simulink model "Lab1"  (Simulink 8.8)
settings: Solver=FixedStepAuto  StartTime=0.0  StopTime=10  FixedStep=0.001  MaxStep=10^-3  RelTol=1e-3  EnableMultiTasking=on
settings Model: Creator=student  LastModifiedBy=Admin
settings OptimizationCC: ExpressionDepthLimit=2147483647  InitFltsAndDblsToZero=on
settings DebuggingCC: SaveWithParameterizedLinksMsg=none  SolverPrmCheckMsg=warning
settings GRTTargetCC: TargetFcnLib=ansi_tfl_tmw.mat  GeneratePreprocessorConditionals=Use local settings

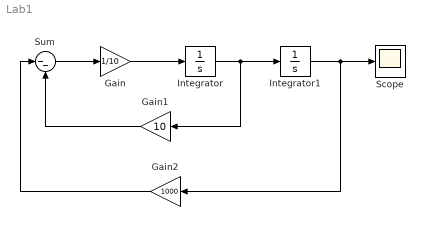
== system Lab1 ==
  Gain : Gain  Gain=1/10
  Gain1 : Gain  Gain=10
  Gain2 : Gain  Gain=1000
  Integrator : Integrator  InitialCondition=1
  Integrator1 : Integrator
  Scope : Scope
  Sum : Sum  Inputs=|--
  wires:
  Sum/1 -> Gain/1
  Gain/1 -> Integrator/1
  Integrator/1 -> Integrator1/1, Gain1/1
  Integrator1/1 -> Scope/1, Gain2/1
  Gain1/1 -> Sum/2
  Gain2/1 -> Sum/1
